simulink library "XPlaneConnect"  (R2019a)
settings: Solver=VariableStepAuto  StartTime=0.0  StopTime=10.0  RelTol=1e-3
settings Model: Creator=simon  LastModifiedBy=simon

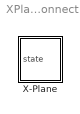
== system XPlaneConnect ==
  X-Plane : MATLAB Function  StartFcn=pauseSimulation  StopFcn=closeSocket  TreatAsAtomicUnit=on

== matlab function XPlaneConnect/X-Plane ==
  data: state input
function updatePOSI(state)
    coder.extrinsic('updateXplanePosition');
    updateXplanePosition(state);
end
